simulink model "ModelMotS_dq"  (R2018b)
settings: Solver=ode45  StartTime=0.0  StopTime=1  MaxStep=1e-4  RelTol=1e-4  EnableMultiTasking=on
values from neighbouring files (symbols this model uses):
  J = 0.045    [gen_sim.m]    (also in gen_sim_new_data_december.m)
  Lfr = 0.007    [gen_sim.m]    (also in gen_sim_new_data_december.m)
  Lfs = 0.007    [gen_sim.m]    (also in gen_sim_new_data_december.m)
  Lmt = 0.210    (= 0.21)    [gen_sim.m]    (also in gen_sim_new_data_december.m)
  Lr = 0.160    (= 0.16)    [gen_sim.m]    (also in gen_sim_new_data_december.m)
  np = 2    [gen_sim.m]    (also in gen_sim_new_data_december.m)
  P1 = 0.7    [gen_sim.m]    (also in gen_sim_new_data_december.m)
  P2 = 1.5    [gen_sim.m]    (also in gen_sim_new_data_december.m)
  Prinit = [ 0 ; 0 ]    [gen_sim.m]    (also in gen_sim_new_data_december.m)
  Psdnom = 0.95    [gen_sim.m]    (also in gen_sim_new_data_december.m)
  Psinit = [ 0 ; 0 ]    [gen_sim.m]    (also in gen_sim_new_data_december.m)
  Rr = 0.9    [gen_sim.m]    (also in gen_sim_new_data_december.m)
  Rs = 1.5    [gen_sim.m]    (also in gen_sim_new_data_december.m)
  tauL = 25    [gen_sim.m]    (also in gen_sim_new_data_december.m)
  thrinit = 0    [gen_sim.m]    (also in gen_sim_new_data_december.m)
  Ts = 0.000250    (= 0.00025)    [gen_sim.m]    (also in gen_sim_new_data_december.m)
  Ulim = 415*sqrt(2/3)    [gen_sim.m]    (also in gen_sim_new_data_december.m)
  Uo = 15    [gen_sim.m]    (also in gen_sim_new_data_december.m)
  wL = 2*pi*0    (= 0)    [gen_sim.m]    (also in gen_sim_new_data_december.m)
  wrinit = 2*pi*0    (= 0)    [gen_sim.m]    (also in gen_sim_new_data_december.m)
libraries: simulink x5
(part 1 of 2)
settings Model: Creator=stbp106  LastModifiedBy=root
settings DataIOCC: LimitDataPoints=on  SaveFormat=Array
settings OptimizationCC: LifeSpan=inf
settings DebuggingCC: UnderspecifiedInitializationDetection=Classic  MergeDetectMultiDrivingBlocksExec=none  SolverPrmCheckMsg=warning  SFUnexpectedBacktrackingDiag=warning  SFNoUnconditionalDefaultTransitionDiag=warning  SFExecutionAtInitializationDiag=none
settings HardwareCC: ProdBitPerPointer=32  ProdBitPerSizeT=32  ProdBitPerPtrDiffT=32  ProdLargestAtomicFloat=None  ProdIntDivRoundTo=Undefined  ProdEndianess=Unspecified  ProdWordSize=32  ProdHWDeviceType=32-bit Generic
settings ModelReferenceCC: PropagateSignalLabelsOutOfModel=off
settings SFSimCC: SimUseLocalCustomCode=off
settings RTWCC: RTWUseLocalCustomCode=off
settings CodeAppCC: StateflowObjectComments=on
settings GRTTargetCC: TargetLangStandard=C89/C90 (ANSI)  GeneratePreprocessorConditionals=Disable all
settings ConfigComp: CovMetricSettings=dw  CovHtmlReporting=on  CovSaveCumulativeToWorkspaceVar=on  CovSaveSingleToWorkspaceVar=on  CovExternalEMLEnable=off  CovSFcnEnable=off

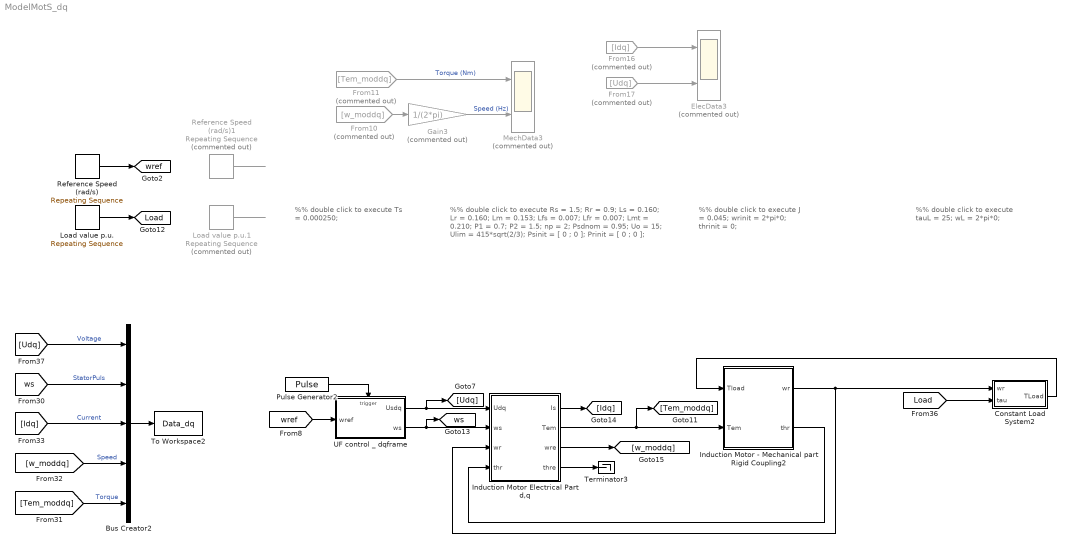
== system ModelMotS_dq ==
  note: %% double click to execute
      |
      | Rs = 1.5; Rr = 0.9;
      | Ls = 0.160; Lr = 0.160; Lm = 0.153;
      | Lfs = 0.007; Lfr = 0.007; Lmt = 0.210; P1 = 0.7; P2 = 1.5;
      | np = 2;
      | Psdnom = 0.95; Uo = 15; Ulim = 415*sqrt(2/3);
      | Psinit = [ 0 ; 0 ]; Prinit = [ 0 ; 0 ];
  note: %% double click to execute
      |
      | J = 0.045;
      | wrinit = 2*pi*0;
      | thrinit = 0;
  note: %% double click to execute
      |
      | tauL = 25;
      | wL = 2*pi*0;
  note: %% double click to execute
      |
      | Ts = 0.000250;
  Bus Creator2 : BusCreator  Inputs=5
  Constant Load System2 : Subsystem  Description=""
  ElecData3 : Scope  Commented=on  NumInputPorts=2
  From10 : From  Commented=on  GotoTag=w_moddq
  From11 : From  Commented=on  GotoTag=Tem_moddq
  From16 : From  Commented=on  GotoTag=Idq
  From17 : From  Commented=on  GotoTag=Udq
  Gain3 : Gain  Commented=on  Gain=1/(2*pi)  SaturateOnIntegerOverflow=on  OutDataTypeStr=Inherit: Same as input  ParamDataTypeStr=Inherit: Same as input
  Induction Motor Electrical Part d,q : Subsystem  Description=""
  Induction Motor - Mechanical part Rigid Coupling2 : Subsystem  Description=""
  Load value p.u. : simulink/Sources/Repeating Sequence  rep_seq_t="[0       0.001       0.002       0.003       0.004       0.005       0.006       0.007       0.008       0.009        0.01       0.011       0.012       0.013       0.014       0.015       0.016       0.017       0.018       0.019        0.02       0.021       0.022       0.023       0.024       0.025       0.026       0.027       0.028       0.029        0.03       0.031       0.032       0.033       0.034       0.035       0.036       0.037       0.038       0.039        0.04       0.041       0.042       0.043       0.044       0.045       0.046       0.047       0.048       0.049        0.05       0.051       0.052       0.053       0.054       0.055       0.056       0.057       0.058       0.059        0.06       0.061       0.062       0.063       0.064       0.065       0.066       0.067       0.068       0.069        0.07       0.071       0.072       0.073       0.074       0.075       0.076       0.077       0.078       0.079        0.08       0.081       0.082       0.083       0.084       0.085       0.086       0.087       0.088       0.089        0.09       0.091       0.092       0.093       0.094       0.095       0.096       0.097       0.098       0.099         0.1       0.101       0.102       0.103       0.104       0.105       0.106       0.107       0.108       0.109        0.11       0.111       0.112       0.113       0.114       0.115       0.116       0.117       0.118       0.119        0.12       0.121       0.122       0.123       0.124       0.125       0.126       0.127       0.128       0.129        0.13       0.131       0.132       0.133       0.134       0.135       0.136       0.137       0.138       0.139        0.14       0.141       0.142       0.143       0.144       0.145       0.146       0.147       0.148       0.149        0.15       0.151       0.152       0.153       0.154       0.155       0.156       0.157       0.158       0.159        0.16       0.161       0.162       0.163       0.164       0.165       0.166       0.167       0.168       0.169        0.17       0.171       0.172       0.173       0.174       0.175       0.176       0.177       0.178       0.179        0.18       0.181       0.182       0.183       0.184       0.185       0.186       0.187       0.188       0.189        0.19       0.191       0.192       0.193       0.194       0.195       0.196       0.197       0.198       0.199         0.2       0.201       0.202       0.203       0.204       0.205       0.206       0.207       0.208       0.209        0.21       0.211       0.212       0.213       0.214       0.215       0.216       0.217       0.218       0.219        0.22       0.221       0.222       0.223       0.224       0.225       0.226       0.227       0.228       0.229        0.23       0.231       0.232       0.233       0.234       0.235       0.236       0.237       0.238       0.239        0.24       0.241       0.242       0.243       0.244       0.245       0.246       0.247       0.248       0.249        0.25       0.251       0.252       0.253       0.254       0.255       0.256       0.257       0.258       0.259        0.26       0.261       0.262       0.263       0.264       0.265       0.266       0.267       0.268       0.269        0.27       0.271       0.272       0.273       0.274       0.275       0.276       0.277       0.278       0.279        0.28       0.281       0.282       0.283       0.284       0.285       0.286       0.287       0.288       0.289        0.29       0.291       0.292       0.293       0.294       0.295       0.296       0.297       0.298       0.299         0.3       0.301       0.302       0.303       0.304       0.305       0.306       0.307       0.308       0.309        0.31       0.311       0.312       0.313       0.314       0.315       0.316       0.317       0.318       0.319        0.32       0.321       0.322       0.323       0.324       0.325       0.326       0.327       0.328       0.329        0.33       0.331       0.332       0.333 ...(+7991 chars)]"  rep_seq_y="[0     0.40028     0.40056     0.40085     0.40113     0.40141     0.40169     0.40197     0.40225     0.40254     0.40282      0.4031     0.40338     0.40366     0.40395     0.40423     0.40451     0.40479     0.40507     0.40535     0.40564     0.40592      0.4062     0.40648     0.40676     0.40705     0.40733     0.40761     0.40789     0.40817     0.40845     0.40874     0.40902      0.4093     0.40958     0.40986     0.41015     0.41043     0.41071     0.41099     0.41127     0.41155     0.41184     0.41212      0.4124     0.41268     0.41296     0.41325     0.41353     0.41381     0.41409     0.41437     0.41465     0.41494     0.41522      0.4155     0.41578     0.41606     0.41635     0.41663     0.41691     0.41719     0.41747     0.41775     0.41804     0.41832      0.4186     0.41888     0.41916     0.41945     0.41973     0.42001     0.42029     0.42057     0.42085     0.42114     0.42142      0.4217     0.42198     0.42226     0.42255     0.42283     0.42311     0.42339     0.42367     0.42396     0.42424     0.42452      0.4248     0.42508     0.42536     0.42565     0.42593     0.42621     0.42649     0.42677     0.42706     0.42734     0.42762      0.4279     0.42818     0.42846     0.42875     0.42903     0.42931     0.42959     0.42987     0.43016     0.43044     0.43072       0.431     0.43128     0.43156     0.43185     0.43213     0.43241     0.43269     0.43297     0.43326     0.43354     0.43382      0.4341     0.43438     0.43466     0.43495     0.43523     0.43551     0.43579     0.43607     0.43636     0.43664     0.43692      0.4372     0.43748     0.43776     0.43805     0.43833     0.43861     0.43889     0.43917     0.43946     0.43974     0.44002      0.4403     0.44058     0.44086     0.44115     0.44143     0.44171     0.44199     0.44227     0.44256     0.44284     0.44312      0.4434     0.44368     0.44396     0.44425     0.44453     0.44481     0.44509     0.44537     0.44566     0.44594     0.44622      0.4465     0.44678     0.44706     0.44735     0.44763     0.44791     0.44819     0.44847     0.44876     0.44904     0.44932      0.4496     0.44988     0.45016     0.45045     0.45073     0.45101     0.45129     0.45157     0.45186     0.45214     0.45242      0.4527     0.45298     0.45326     0.45355     0.45383     0.45411     0.45439     0.45467     0.45496     0.45524     0.45552      0.4558     0.45608     0.45636     0.45665     0.45693     0.45721     0.45749     0.45777     0.45806     0.45834     0.45862      0.4589     0.45918     0.45946     0.45975     0.46003     0.46031     0.46059     0.46087     0.46116     0.46144     0.46172       0.462     0.46228     0.46256     0.46285     0.46313     0.46341     0.46369     0.46397     0.46426     0.46454     0.46482      0.4651     0.46538     0.46567     0.46595     0.46623     0.46651     0.46679     0.46707     0.46736     0.46764     0.46792      0.4682     0.46848     0.46877     0.46905     0.46933     0.46961     0.46989     0.47017     0.47046     0.47074     0.47102      0.4713     0.47158     0.47187     0.47215     0.47243     0.47271     0.47299     0.47327     0.47356     0.47384     0.47412      0.4744     0.47468     0.47497     0.47525     0.47553     0.47581     0.47609     0.47637     0.47666     0.47694     0.47722      0.4775     0.47778     0.47807     0.47835     0.47863     0.47891     0.47919     0.47947     0.47976     0.48004     0.48032      0.4806     0.48088     0.48117     0.48145     0.48173     0.48201     0.48229     0.48257     0.48286     0.48314     0.48342      0.4837     0.48398     0.48427     0.48455     0.48483     0.48511     0.48539     0.48567     0.48596     0.48624     0.48652      0.4868     0.48708     0.48737     0.48765     0.48793     0.48821     0.48849     0.48877     0.48906     0.48934     0.48962      0.4899     0.49018     0.49047     0.49075     0.49103     0.49131     0.49159     0.49187     0.49216     0.49244     0.49272       0.493     0.49328     0.49357     0.49385 ...(+7991 chars)]"
  Load value p.u.1 : simulink/Sources/Repeating Sequence  Commented=on  rep_seq_t=[ 0 4 8 9 11 12 12.5 100 ]  rep_seq_y="[0 0 2 2 0  0 1 1]"
  MechData3 : Scope  Commented=on  NumInputPorts=2
  Pulse Generator2 : DiscretePulseGenerator  PulseType=Time based  Period=Ts  PulseWidth=50
  Reference Speed (rad/s) : simulink/Sources/Repeating Sequence  rep_seq_t="[0       0.001       0.002       0.003       0.004       0.005       0.006       0.007       0.008       0.009        0.01       0.011       0.012       0.013       0.014       0.015       0.016       0.017       0.018       0.019        0.02       0.021       0.022       0.023       0.024       0.025       0.026       0.027       0.028       0.029        0.03       0.031       0.032       0.033       0.034       0.035       0.036       0.037       0.038       0.039        0.04       0.041       0.042       0.043       0.044       0.045       0.046       0.047       0.048       0.049        0.05       0.051       0.052       0.053       0.054       0.055       0.056       0.057       0.058       0.059        0.06       0.061       0.062       0.063       0.064       0.065       0.066       0.067       0.068       0.069        0.07       0.071       0.072       0.073       0.074       0.075       0.076       0.077       0.078       0.079        0.08       0.081       0.082       0.083       0.084       0.085       0.086       0.087       0.088       0.089        0.09       0.091       0.092       0.093       0.094       0.095       0.096       0.097       0.098       0.099         0.1       0.101       0.102       0.103       0.104       0.105       0.106       0.107       0.108       0.109        0.11       0.111       0.112       0.113       0.114       0.115       0.116       0.117       0.118       0.119        0.12       0.121       0.122       0.123       0.124       0.125       0.126       0.127       0.128       0.129        0.13       0.131       0.132       0.133       0.134       0.135       0.136       0.137       0.138       0.139        0.14       0.141       0.142       0.143       0.144       0.145       0.146       0.147       0.148       0.149        0.15       0.151       0.152       0.153       0.154       0.155       0.156       0.157       0.158       0.159        0.16       0.161       0.162       0.163       0.164       0.165       0.166       0.167       0.168       0.169        0.17       0.171       0.172       0.173       0.174       0.175       0.176       0.177       0.178       0.179        0.18       0.181       0.182       0.183       0.184       0.185       0.186       0.187       0.188       0.189        0.19       0.191       0.192       0.193       0.194       0.195       0.196       0.197       0.198       0.199         0.2       0.201       0.202       0.203       0.204       0.205       0.206       0.207       0.208       0.209        0.21       0.211       0.212       0.213       0.214       0.215       0.216       0.217       0.218       0.219        0.22       0.221       0.222       0.223       0.224       0.225       0.226       0.227       0.228       0.229        0.23       0.231       0.232       0.233       0.234       0.235       0.236       0.237       0.238       0.239        0.24       0.241       0.242       0.243       0.244       0.245       0.246       0.247       0.248       0.249        0.25       0.251       0.252       0.253       0.254       0.255       0.256       0.257       0.258       0.259        0.26       0.261       0.262       0.263       0.264       0.265       0.266       0.267       0.268       0.269        0.27       0.271       0.272       0.273       0.274       0.275       0.276       0.277       0.278       0.279        0.28       0.281       0.282       0.283       0.284       0.285       0.286       0.287       0.288       0.289        0.29       0.291       0.292       0.293       0.294       0.295       0.296       0.297       0.298       0.299         0.3       0.301       0.302       0.303       0.304       0.305       0.306       0.307       0.308       0.309        0.31       0.311       0.312       0.313       0.314       0.315       0.316       0.317       0.318       0.319        0.32       0.321       0.322       0.323       0.324       0.325       0.326       0.327       0.328       0.329        0.33       0.331       0.332       0.333 ...(+7991 chars)]"  rep_seq_y="[0  0.00023815  0.00047629  0.00071444  0.00095259   0.0011907   0.0014289    0.001667   0.0019052   0.0021433   0.0023815   0.0026196   0.0028578   0.0030959   0.0033341   0.0035722   0.0038103   0.0040485   0.0042866   0.0045248   0.0047629   0.0050011   0.0052392   0.0054774   0.0057155   0.0059537   0.0061918     0.00643   0.0066681   0.0069063   0.0071444   0.0073826   0.0076207   0.0078588    0.008097   0.0083351   0.0085733   0.0088114   0.0090496   0.0092877   0.0095259    0.009764    0.010002     0.01024    0.010478    0.010717    0.010955    0.011193    0.011431    0.011669    0.011907    0.012145    0.012384    0.012622     0.01286    0.013098    0.013336    0.013574    0.013813    0.014051    0.014289    0.014527    0.014765    0.015003    0.015241     0.01548    0.015718    0.015956    0.016194    0.016432     0.01667    0.016908    0.017147    0.017385    0.017623    0.017861    0.018099    0.018337    0.018575    0.018814    0.019052     0.01929    0.019528    0.019766    0.020004    0.020242    0.020481    0.020719    0.020957    0.021195    0.021433    0.021671     0.02191    0.022148    0.022386    0.022624    0.022862      0.0231    0.023338    0.023577    0.023815    0.024053    0.024291    0.024529    0.024767    0.025005    0.025244    0.025482     0.02572    0.025958    0.026196    0.026434    0.026672    0.026911    0.027149    0.027387    0.027625    0.027863    0.028101    0.028339    0.028578    0.028816    0.029054    0.029292     0.02953    0.029768    0.030007    0.030245    0.030483    0.030721    0.030959    0.031197    0.031435    0.031674    0.031912     0.03215    0.032388    0.032626    0.032864    0.033102    0.033341    0.033579    0.033817    0.034055    0.034293    0.034531    0.034769    0.035008    0.035246    0.035484    0.035722     0.03596    0.036198    0.036436    0.036675    0.036913    0.037151    0.037389    0.037627    0.037865    0.038103    0.038342     0.03858    0.038818    0.039056    0.039294    0.039532    0.039771    0.040009    0.040247    0.040485    0.040723    0.040961    0.041199    0.041438    0.041676    0.041914    0.042152     0.04239    0.042628    0.042866    0.043105    0.043343    0.043581    0.043819    0.044057    0.044295    0.044533    0.044772     0.04501    0.045248    0.045486    0.045724    0.045962      0.0462    0.046439    0.046677    0.046915    0.047153    0.047391    0.047629    0.047868    0.048106    0.048344    0.048582     0.04882    0.049058    0.049296    0.049535    0.049773    0.050011    0.050249    0.050487    0.050725    0.050963    0.051202     0.05144    0.051678    0.051916    0.052154    0.052392     0.05263    0.052869    0.053107    0.053345    0.053583    0.053821    0.054059    0.054297    0.054536    0.054774    0.055012     0.05525    0.055488    0.055726    0.055965    0.056203    0.056441    0.056679    0.056917    0.057155    0.057393    0.057632     0.05787    0.058108    0.058346    0.058584    0.058822     0.05906    0.059299    0.059537    0.059775    0.060013    0.060251    0.060489    0.060727    0.060966    0.061204    0.061442     0.06168    0.061918    0.062156    0.062394    0.062633    0.062871    0.063109    0.063347    0.063585    0.063823    0.064062      0.0643    0.064538    0.064776    0.065014    0.065252     0.06549    0.065729    0.065967    0.066205    0.066443    0.066681    0.066919    0.067157    0.067396    0.067634    0.067872     0.06811    0.068348    0.068586    0.068824    0.069063    0.069301    0.069539    0.069777    0.070015    0.070253    0.070491     0.07073    0.070968    0.071206    0.071444    0.071682     0.07192    0.072158    0.072397    0.072635    0.072873    0.073111    0.073349    0.073587    0.073826    0.074064    0.074302     0.07454    0.074778    0.075016    0.075254    0.075493    0.075731    0.075969    0.076207    0.076445    0.076683    0.076921     0.07716    0.077398    0.077636    0.077874    0.078112     0.07835    0.078588    0.078827    0.079065    0.079303 ...(+7991 chars)]"
  Reference Speed (rad/s)1 : simulink/Sources/Repeating Sequence  Commented=on  rep_seq_t="[ 0 3 14 15 16  17 18 19 100 ]"  rep_seq_y="[0 1 1  0.5  0.5  1.2 1.2  1 1]*2*pi*50"
  Terminator3 : Terminator
  To Workspace2 : ToWorkspace  VariableName=Data_dq  SaveFormat=Timeseries  SampleTime=-1
  UF control _ dqframe : Subsystem
  tag scope: Load=global, wref=global, ws=global
  wires:
  Reference Speed (rad/s)/1 -> [wref]
  Induction Motor - Mechanical part Rigid Coupling2/2(thr) -> Induction Motor Electrical Part d,q/4(thr)
  Induction Motor Electrical Part d,q/2(Tem) -> [Tem_moddq], Induction Motor - Mechanical part Rigid Coupling2/2(Tem)
  Induction Motor - Mechanical part Rigid Coupling2/1(wr) -> Induction Motor Electrical Part d,q/3(wr), Constant Load System2/1(wr)
  Induction Motor Electrical Part d,q/4(thre) -> Terminator3/1
  Constant Load System2/1(TLoad) -> Induction Motor - Mechanical part Rigid Coupling2/1(Tload)
  Induction Motor Electrical Part d,q/1(Is) -> [Idq]
  Induction Motor Electrical Part d,q/3(wre) -> [w_moddq]
  [Load] -> Constant Load System2/2(tau)
  UF control _ dqframe/1(Usdq) -> [Udq], Induction Motor Electrical Part d,q/1(Udq)
  Pulse Generator2/1 -> UF control _ dqframe/Trigger
  UF control _ dqframe/2(ws) -> [ws], Induction Motor Electrical Part d,q/2(ws)
  [wref] -> UF control _ dqframe/1(wref)
  From16/1 -> ElecData3/1
  From17/1 -> ElecData3/2
  From10/1 -> Gain3/1
  From11/1 -> MechData3/1  "Torque (Nm)"
  Gain3/1 -> MechData3/2  "Speed (Hz)"
  Load value p.u./1 -> [Load]
  [Udq] -> Bus Creator2/1  "Voltage"
  [Idq] -> Bus Creator2/3  "Current"
  [w_moddq] -> Bus Creator2/4  "Speed"
  [Tem_moddq] -> Bus Creator2/5  "Torque"
  Bus Creator2/1 -> To Workspace2/1
  [ws] -> Bus Creator2/2  "StatorPuls"
  Reference Speed (rad/s)1/1 -> ?
  Load value p.u.1/1 -> ?
